simulink model "useCaseMDL_ros"  (R2024b)
settings: Solver=FixedStepAuto  StartTime=0.0  StopTime=10.0  RelTol=1e-3
model workspace (MAT data in the model file):
  SL_ROS_VariableLengthArrays_MaxSizes.CommonInfo.ArrayTruncateAction = 'EmitWarning'
  SL_ROS_VariableLengthArrays_MaxSizes.MsgTypeMap = containers.Map
  SL_ROS_VariableLengthArrays_MaxSizes.MsgTypeMap.serialization.keys = {'std_msgs/Float32MultiArray', 'std_msgs/Float64MultiArray'}
  SL_ROS_VariableLengthArrays_MaxSizes.MsgTypeMap.serialization.values{1}.PropertyName = 'data'
  SL_ROS_VariableLengthArrays_MaxSizes.MsgTypeMap.serialization.values{1}.DataType = 'single'
  SL_ROS_VariableLengthArrays_MaxSizes.MsgTypeMap.serialization.values{1}.MaxLength = 1500000
  SL_ROS_VariableLengthArrays_MaxSizes.MsgTypeMap.serialization.values{2}.PropertyName = 'data'
  SL_ROS_VariableLengthArrays_MaxSizes.MsgTypeMap.serialization.values{2}.DataType = 'double'
  SL_ROS_VariableLengthArrays_MaxSizes.MsgTypeMap.serialization.values{2}.MaxLength = 30000
  SL_ROS_VariableLengthArrays_MaxSizes.MsgTypeMap.serialization.uniformity = 0
  SL_ROS_VariableLengthArrays_MaxSizes.MsgTypeMap.serialization.keyType = 'char'
  SL_ROS_VariableLengthArrays_MaxSizes.MsgTypeMap.serialization.valueType = 'any'
undefined symbols (not defined in the file or in its folder): dem, gridLoc, originalReferencePath, res
libraries: roshelperlib x9, commrandsrc3 x1, dspstat3 x1
settings Model: DataDictionary=ros2lib.sldd  Creator=cstabile  LastModifiedBy=jbrault
settings SolverCC: DateTimeAtSimulationTimeZero=[]
settings OptimizationCC: EnhancedBackFolding=on  PassReuseOutputArgsAs=Individual arguments  ZeroExternalMemoryAtStartup=off  ZeroInternalMemoryAtStartup=off  MaxStackSize=64  OptimizeBlockOrder=speed  DifferentSizesBufferReuse=on  OptimizationCustomize=off  EfficientTunableParamExpr=on
settings DebuggingCC: ParameterTunabilityLossMsg=error
settings SFSimCC: MATLABDynamicMemAlloc=off
settings RTWCC: Description=Embedded Coder  SystemTargetFile=ert.tlc  HardwareBoard=Robot Operating System 2 (ROS 2)  TLCOptions="-aInlineSetEventsForThisBaseRateFcn=TLC_FALSE -aSuppressMultiTaskScheduler=TLC_FALSE  -aRateBasedStepFcn=0"  TemplateMakefile=ert_default_tmf  Toolchain=Colcon Tools  TargetLang=C++
settings CodeAppCC: ForceParamTrailComments=on  IgnoreCustomStorageClasses=off  OperatorAnnotations=on  SimulinkDataObjDesc=on  SFDataObjDesc=on  InsertBlockDesc=on
settings ERTTargetCC: CodeInterfacePackaging=C++ class  InlinedParameterPlacement=Hierarchical  RootIOFormat=Structure reference  DynamicArrayContainerType=coder::array

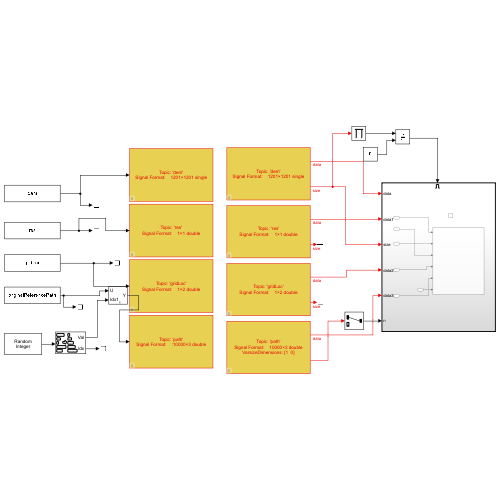
[thumbnail: Simulink's stored preview of the top-level diagram]
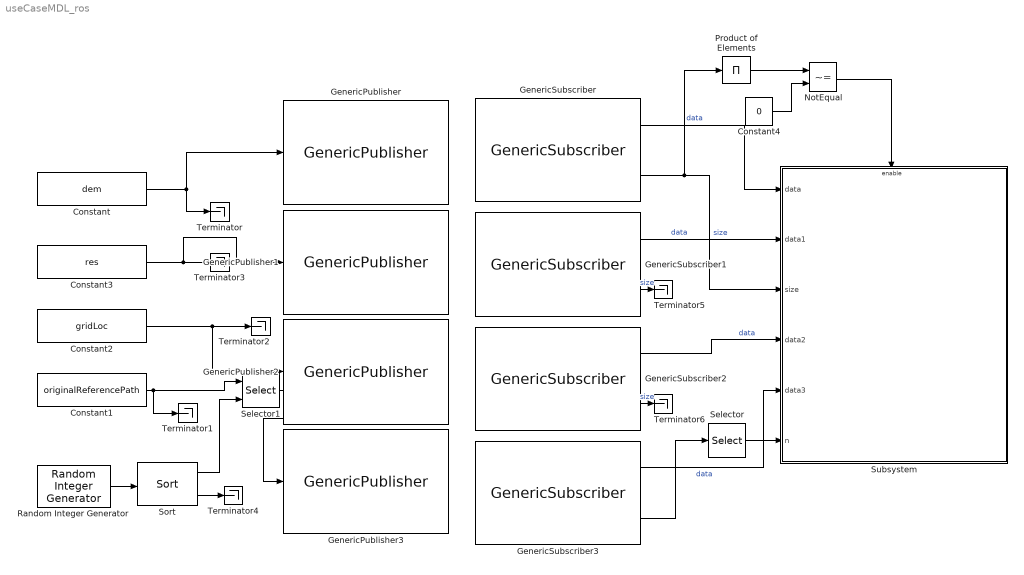
== system useCaseMDL_ros ==
  Constant : Constant  Value=dem  VectorParams1D=off
  Constant1 : Constant  Value=originalReferencePath  VectorParams1D=off
  Constant2 : Constant  Value=gridLoc
  Constant3 : Constant  Value=res
  Constant4 : Constant  Value=0
  GenericPublisher : roshelperlib/GenericPublisher  userDataType=single  dims=[1201 1201]  topicName='dem'  isVarsize=off  varsizeDims=[1 0]
  GenericPublisher1 : roshelperlib/GenericPublisher  userDataType=double  dims=[1 1]  topicName='res'  isVarsize=off  varsizeDims=[1 0]
  GenericPublisher2 : roshelperlib/GenericPublisher  userDataType=double  dims=[1 2]  topicName='gridLoc'  isVarsize=off  varsizeDims=[1 0]
  GenericPublisher3 : roshelperlib/GenericPublisher  userDataType=double  dims=[1e4 3]  topicName='path'  isVarsize=on  varsizeDims=[1 0]
  GenericSubscriber : roshelperlib/GenericSubscriber  userDataType=single  dims=[1201 1201]  topicName='dem'  isVarsize=off  varsizeDims=[1 0]  returnFixedTF=off
  GenericSubscriber1 : roshelperlib/GenericSubscriber  userDataType=double  dims=[1 1]  topicName='res'  isVarsize=off  varsizeDims=[1 0]  returnFixedTF=off
  GenericSubscriber2 : roshelperlib/GenericSubscriber  userDataType=double  dims=[1 2]  topicName='gridLoc'  isVarsize=off  varsizeDims=[1 0]  returnFixedTF=off
  GenericSubscriber3 : roshelperlib/GenericSubscriber  userDataType=double  dims=[1e4 3]  topicName='path'  isVarsize=on  varsizeDims=[1 0]  returnFixedTF=on
  NotEqual : RelationalOperator  Operator=~=  OutDataTypeStr=boolean  RndMeth=Simplest  InputSameDT=off
  Product of Elements : Product  Inputs=*
  Random Integer Generator : commrandsrc3/Random Integer Generator  SetSize=3000  SeedSource=Auto  Seed=0  SampleTime=1  SamplesPerFrame=2  OutputDataType=double  SimulateUsing=Interpreted execution
  Selector : Selector  InputPortWidth=2  IndexOptions=Index vector (dialog)  Indices=1  OutputSizes=1
  Selector1 : Selector  NumberOfDimensions=2  InputPortWidth=3  IndexOptions=Starting and ending indices (port),Select all  Indices=[1 3],1  OutputSizes=1,1
  Sort : dspstat3/Sort  otype=Value and Index  dir=Ascending  sortAlg=Quick sort  roundingMode=Floor  overflowMode=off  accumDataTypeStr=Inherit: Same as product output  accumLastDataTypeStr=Inherit: Same as product output
  Subsystem : Subsystem
  Terminator{,1..6} (7 alike) : Terminator
  wires:
  Constant1/1 -> Selector1/1, Terminator1/1
  GenericSubscriber3/2 -> Selector/1
  Constant3/1 -> GenericPublisher1/1, Terminator3/1
  Constant/1 -> Terminator/1, GenericPublisher/1
  Constant2/1 -> GenericPublisher2/1, Terminator2/1
  Random Integer Generator/1 -> Sort/1
  Sort/1 -> Selector1/2
  Sort/2 -> Terminator4/1
  Selector1/1 -> GenericPublisher3/1
  GenericSubscriber1/2 -> Terminator5/1  "size"
  GenericSubscriber2/2 -> Terminator6/1  "size"
  GenericSubscriber/1 -> Subsystem/1(data)  "data"
  GenericSubscriber1/1 -> Subsystem/2(data1)  "data"
  GenericSubscriber/2 -> Product of Elements/1, Subsystem/3(size)  "size"
  GenericSubscriber2/1 -> Subsystem/4(data2)  "data"
  GenericSubscriber3/1 -> Subsystem/5(data3)  "data"
  Selector/1 -> Subsystem/6(n)
  Product of Elements/1 -> NotEqual/1
  Constant4/1 -> NotEqual/2
  NotEqual/1 -> Subsystem/Enable

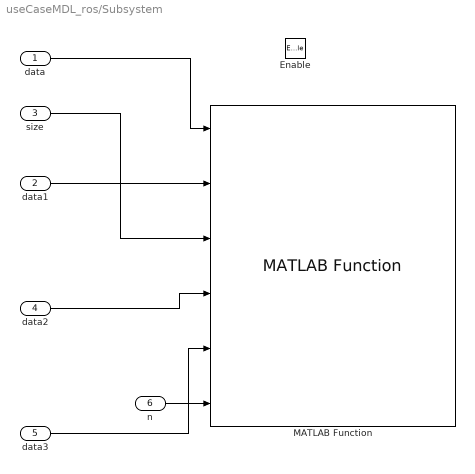
== system useCaseMDL_ros/Subsystem ==
  data : Inport
  data1 : Inport  Port=2
  size : Inport  Port=3
  data2 : Inport  Port=4
  data3 : Inport  Port=5
  n : Inport  Port=6
  Enable : EnablePort
  MATLAB Function : roshelperlib/MATLAB Function  mapType="\"Generic\""
  wires:
  data2/1 -> MATLAB Function/4
  data3/1 -> MATLAB Function/5
  data1/1 -> MATLAB Function/2
  data/1 -> MATLAB Function/1
  size/1 -> MATLAB Function/3
  n/1 -> MATLAB Function/6
